simulink model "Plastic_Washer_R2020a"  (R2020a)
settings: Solver=VariableStepAuto  StartTime=0.0  StopTime=60*60*8  RelTol=1e-3  AbsTol=1e-3
libraries: fl_lib x20, nesl_utility x7, simulink x2, SimscapeFluids_lib x1
settings Model: Creator=YXL1108  LastModifiedBy=YXL1108
settings SolverCC: AutoScaleAbsTol=off
settings DebuggingCC: SymbolicDimsDataTypeCodeGenerationDiagnostic=none
settings SFSimCC: CustomCodeUndefinedFunction=UseInterfaceOnly
settings SimscapeCC: SimscapeLogType=all  SimscapeLogSimulationStatistics=on  SimscapeLogDataHistory=10000

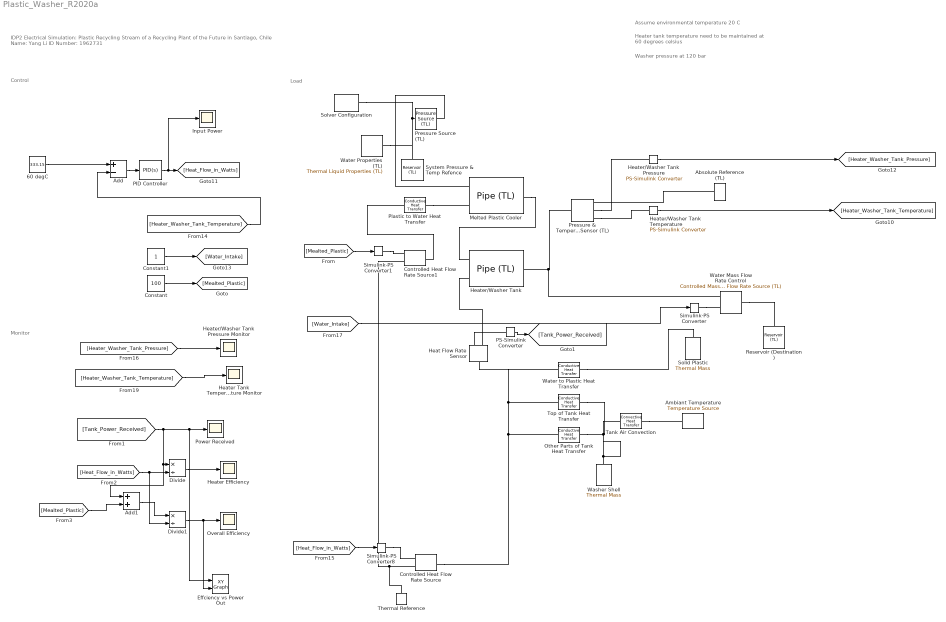
== system Plastic_Washer_R2020a ==
  note: Washer pressure at 120 bar
  note: Load
  note: Monitor
  note: Control
  note: Heater tank temperature need to be maintained at
      | 60 degrees celsius
  note: Assume environmental temperature 20 C
  note: IDP2 Electrical Simulation: Plastic Recycling Stream of a Recycling Plant of the Future in Santiago, Chile
      | Name: Yang Li
      | ID Number: 1962731
  60 degC : Constant  Value=333.15
  Absolute Reference (TL) : fl_lib/Thermal Liquid/Elements/Absolute Reference (TL)
      settings: SourceProductBaseCode=SS
  Add : Sum  Inputs=+-
  Add1 : Sum
  Ambiant Temperature : fl_lib/Thermal/Thermal Sources/Temperature Source  temperature=20 degC
  Constant : Constant  Value=100
  Constant1 : Constant
  Controlled Heat Flow Rate Source : fl_lib/Thermal/Thermal Sources/Controlled Heat Flow Rate Source
  Controlled Heat Flow Rate Source1 : fl_lib/Thermal/Thermal Sources/Controlled Heat Flow Rate Source
  Divide : Product  Inputs=*/
  Divide1 : Product  Inputs=*/
  Effciency vs Power Out : simulink/Sinks/XY Graph  xmin=1.63e+5  xmax=1.645e+5  ymin=0  ymax=1  st=-1
  Heat Flow Rate Sensor : fl_lib/Thermal/Thermal Sensors/Heat Flow Rate Sensor
      settings: SourceProductBaseCode=SS
  Heater Efficiency : Scope
  Heater Tank Temperature Monitor : Scope
  Heater/Washer Tank : fl_lib/Thermal Liquid/Elements/Pipe (TL)  length=3.5 m  area=12.25 m^2  Dh=3.5 m  length_add=1 m  roughness=15e-6 m  Re_lam=2000  Re_tur=4000  shape_factor=64  Nu_lam=3.66  dynamic_compressibility=simscape.enum.onoff.on  inertia=simscape.enum.onoff.off  p0=1 bar  T0=20 degC  mdot0=0 kg/s
      settings: SourceProductBaseCode=SS
  Heater/Washer Tank Pressure : nesl_utility/PS-Simulink Converter  PhysicalDomain=network_engine_domain  SubClassName=ps_output  LeftPortType=input  RightPortType=output  PseudoPeriodic=off  Frequencies=[]  Unit=inherit  AffineConversion=off
  Heater/Washer Tank Pressure Monitor : Scope
  Heater/Washer Tank Temperature : nesl_utility/PS-Simulink Converter  PhysicalDomain=network_engine_domain  SubClassName=ps_output  LeftPortType=input  RightPortType=output  PseudoPeriodic=off  Frequencies=[]  Unit=inherit  AffineConversion=off
  Input Power : Scope
  Melted Plastic Cooler : fl_lib/Thermal Liquid/Elements/Pipe (TL)  length=100 m  area=0.0009 m^2  Dh=0.03 m  length_add=1 m  roughness=15e-6 m  Re_lam=2000  Re_tur=4000  shape_factor=64  Nu_lam=3.66  dynamic_compressibility=simscape.enum.onoff.on  inertia=simscape.enum.onoff.off  p0=1 bar  T0=20 degC  mdot0=0 kg/s
      settings: SourceProductBaseCode=SS
  Other Parts of Tank Heat Transfer : fl_lib/Thermal/Thermal Elements/Conductive Heat Transfer  area=40 m^2  thickness=0.05 m  th_cond=45 W/(m*K)  T_specify=off  T_priority=None  T=0 K  T_nominal_specify=off  T_nominal_unit=K  T_nominal_value=1  Q_specify=off  Q_priority=None  Q=0 W  Q_nominal_specify=off  Q_nominal_unit=W  Q_nominal_value=1
  Overall Efficiency : Scope
  PID Controller : simulink/Continuous/PID Controller  Controller=PID  Form=Parallel  TimeDomain=Continuous-time  UseExternalTs=off  SampleTime=-1  IntegratorMethod=Forward Euler  FilterMethod=Forward Euler  ControllerParametersSource=internal  P=10000  I=4  D=1000000000000  UseFilter=on  N=100  TunerSelectOption=Transfer Function Based (PID Tuner App)  InitialConditionSource=internal  InitialConditionForIntegrator=0  InitialConditionForFilter=0  DifferentiatorICPrevScaledInput=0  ExternalReset=none  TrackingMode=off  Kt=1  LimitOutput=off  UpperSaturationLimit=inf  LowerSaturationLimit=-inf  LinearizeAsGain=on  AntiWindupMode=none  Kb=1  POutMin=[]  POutMax=[]  IOutMin=[]  IOutMax=[]  DOutMin=[]  DOutMax=[]  NOutMin=[]  NOutMax=[]  SumOutMin=[]  SumOutMax=[]  SaturationOutMin=[]  SaturationOutMax=[]  PParamMin=[]  PParamMax=[]  IParamMin=[]  IParamMax=[]  DParamMin=[]  DParamMax=[]  NParamMin=[]  NParamMax=[]  KbParamMin=[]  KbParamMax=[]  KtParamMin=[]  KtParamMax=[]  KbOutMin=[]  KbOutMax=[]  KtOutMin=[]  KtOutMax=[]  IntegratorOutMin=[]  IntegratorOutMax=[]  FilterOutMin=[]  FilterOutMax=[]  SumI1OutMin=[]  SumI1OutMax=[]  SumI2OutMin=[]  SumI2OutMax=[]  SumI3OutMin=[]  SumI3OutMax=[]  SumI4OutMin=[]  SumI4OutMax=[]  SumDOutMin=[]  SumDOutMax=[]  DifferentiatorOutMin=[]  DifferentiatorOutMax=[]  FilterDiffOutCoefMin=[]  FilterDiffOutCoefMax=[]  ReciprocalOutMin=[]  ReciprocalOutMax=[]  SumDenOutMin=[]  SumDenOutMax=[]  SumNumOutMin=[]  SumNumOutMax=[]  DivideOutMin=[]  DivideOutMax=[]  UdiffTsProdOutMin=[]  UdiffTsProdOutMax=[]  NTsProdOutMin=[]  NTsProdOutMax=[]  UintegralTsProdOutMin=[]  UintegralTsProdOutMax=[]  UngainTsProdOutMin=[]  UngainTsProdOutMax=[]  IntegratorContinuousStateAttributes=''  IntegratorStateMustResolveToSignalObject=off  IntegratorRTWStateStorageClass=Auto  FilterContinuousStateAttributes=''  FilterStateMustResolveToSignalObject=off  FilterRTWStateStorageClass=Auto  ParallelPVariant=InternalParameters  IdealPVariant=Disabled  IVariant=InternalParameters  DVariant=InternalParameters  IntegratorVariant=Continuous  SatVariant=Disabled  AWVariant=Passthrough  PCopyVariant=Disabled  TRVariant=Disabled  FdbkBlocksVariant=Forward  IdealPFdbkVariant=Disabled  SatFdbkVariant=Disabled  DerivativeFilterVariant=ContFilter  NVariant=InternalParameters  NCopyVariant=Disabled  FilterICVariant=InternalICsFilter  IntegratorICVariant=InternalICs  ExternalResetVariant=Disabled  TRSumVariant=Passthrough  SumFdbkVariant=Disabled  SumVariant=Sum_PID  TsampFilterVariant=InternalTs  TsampNgainVariant=Passthrough  TsampIntegralVariant=Passthrough
  PS-Simulink Converter : nesl_utility/PS-Simulink Converter  PhysicalDomain=network_engine_domain  SubClassName=ps_output  LeftPortType=input  RightPortType=output  PseudoPeriodic=off  Frequencies=[]  Unit=inherit  AffineConversion=off
  Plastic to Water Heat Transfer : fl_lib/Thermal/Thermal Elements/Conductive Heat Transfer  area=12 m^2  thickness=0.1 m  th_cond=401 W/(m*K)  T_specify=off  T_priority=None  T=0 K  T_nominal_specify=off  T_nominal_unit=K  T_nominal_value=1  Q_specify=off  Q_priority=None  Q=0 W  Q_nominal_specify=off  Q_nominal_unit=W  Q_nominal_value=1
  Power Received : Scope
  Pressure & Temperature Sensor (TL) : fl_lib/Thermal Liquid/Sensors/Pressure & Temperature Sensor (TL)
      settings: SourceProductBaseCode=SS  InternalSimscapePortConfiguration="{\"Bottom\":[],\"Left\":[{\"id\":\"A\",\"label\":\"A\",\"type\":\"foundation.thermal_liquid.thermal_liquid\"}],\"Right\":[{\"id\":\"B\",\"label\":\"B\",\"type\":\"foundation.thermal_liquid.thermal_liquid\"},{\"id\":\"P\",\"label\":\"P\",\"type\":\"output\"},{\"id\":\"T\",\"label\":\"T\",\"type\":\"output\"}],\"Top\":[]}"
  Pressure Source (TL) : fl_lib/Thermal Liquid/Sources/Pressure Source (TL)  commanded_pressure=120 bar  area=0.01 m^2
      settings: SourceProductBaseCode=SS  InternalSimscapePortConfiguration="{\"Bottom\":[],\"Left\":[{\"id\":\"A\",\"label\":\"A\",\"type\":\"foundation.thermal_liquid.thermal_liquid\"}],\"Right\":[{\"id\":\"B\",\"label\":\"B\",\"type\":\"foundation.thermal_liquid.thermal_liquid\"}],\"Top\":[]}"
  Reservoir (Destination) : fl_lib/Thermal Liquid/Elements/Reservoir (TL)  pressure_spec=foundation.enum.pressure_spec.atmospheric  reservoir_pressure=0.101325 MPa  reservoir_temperature=20 degC  area=0.01 m^2
      settings: SourceProductBaseCode=SS
  Simulink-PS Converter : nesl_utility/Simulink-PS Converter  PhysicalDomain=network_engine_domain  SubClassName=ps_input  LeftPortType=input  RightPortType=output  PseudoPeriodic=off  Frequencies=[]  NoiseDistribution=none  NoiseParameters=[]  Unit=1  AffineConversion=off  FilteringAndDerivatives=provide  SimscapeFilterOrder=1  InputFilterTimeConstant=0.001  UdotUserProvided=0
  Simulink-PS Converter1 : nesl_utility/Simulink-PS Converter  PhysicalDomain=network_engine_domain  SubClassName=ps_input  LeftPortType=input  RightPortType=output  PseudoPeriodic=off  Frequencies=[]  NoiseDistribution=none  NoiseParameters=[]  Unit=1  AffineConversion=off  FilteringAndDerivatives=provide  SimscapeFilterOrder=1  InputFilterTimeConstant=0.001  UdotUserProvided=0
  Simulink-PS Converter8 : nesl_utility/Simulink-PS Converter  PhysicalDomain=network_engine_domain  SubClassName=ps_input  LeftPortType=input  RightPortType=output  PseudoPeriodic=off  Frequencies=[]  NoiseDistribution=none  NoiseParameters=[]  Unit=1  AffineConversion=off  FilteringAndDerivatives=provide  SimscapeFilterOrder=1  InputFilterTimeConstant=0.001  UdotUserProvided=0
  Solid Plastic : fl_lib/Thermal/Thermal Elements/Thermal Mass  mass=10000 kg  sp_heat=1670 J/kg/K  T_specify=off  T_priority=High  T=300 K  T_nominal_specify=off  T_nominal_unit=K  T_nominal_value=1  Q_specify=off  Q_priority=None  Q=0 W  Q_nominal_specify=off  Q_nominal_unit=W  Q_nominal_value=1
  Solver Configuration : nesl_utility/Solver Configuration  PhysicalDomain=network_engine_domain  SubClassName=solver  LeftPortType=input  RightPortType=generic  Tones=[]  Harmonics=[]  SimulateNoise=off  Profile=off  UseLocalSampling=off  EnableSwitchedLinearOptims=on  FrequencyDomain=off  UseCCode=off  RelTol=0.001  AbsTol=1e-06  MinStep=1e-09  ToWorkspace=off  RevertToSquareIcSolve=off  NumHomotopyIterations=100  PhasorMode=off  PhasorModeNumHarmonics=1  DoDC=off  ResidualTolerance=1e-09  UseLocalSolver=off  LocalSolverChoice=NE_BACKWARD_EULER_ADVANCER  LocalSolverSampleTime=0.001  DoFixedCost=off  MaxNonlinIter=3  MaxModeIter=2  LinearAlgebra=auto  EquationFormulation=NE_TIME_EF  DelaysMemoryBudget=1024  AutomaticFiltering=on  FilteringTimeConstant=0.001  PartitionStorageMethod=AS_NEEDED  PartitionMemoryBudget=1024  PartitionMethod=ROBUST
  System Pressure & Temp Refence : fl_lib/Thermal Liquid/Elements/Reservoir (TL)  pressure_spec=foundation.enum.pressure_spec.atmospheric  reservoir_pressure=0.101325 MPa  reservoir_temperature=20 degC  area=0.01 m^2
      settings: SourceProductBaseCode=SS
  Tank Air Convection : fl_lib/Thermal/Thermal Elements/Convective Heat Transfer  area=48 m^2  heat_tr_coeff=7.9 W/(m^2 * K)  T_specify=off  T_priority=None  T=0 K  T_nominal_specify=off  T_nominal_unit=K  T_nominal_value=1  Q_specify=off  Q_priority=None  Q=0 W  Q_nominal_specify=off  Q_nominal_unit=W  Q_nominal_value=1
  Thermal Reference : fl_lib/Thermal/Thermal Elements/Thermal Reference
  Top of Tank Heat Transfer : fl_lib/Thermal/Thermal Elements/Conductive Heat Transfer  area=8 m^2  thickness=0.05 m  th_cond=60 W/(m*K)  T_specify=off  T_priority=None  T=0 K  T_nominal_specify=off  T_nominal_unit=K  T_nominal_value=1  Q_specify=off  Q_priority=None  Q=0 W  Q_nominal_specify=off  Q_nominal_unit=W  Q_nominal_value=1
  Washer Shell : fl_lib/Thermal/Thermal Elements/Thermal Mass  mass=948 kg  sp_heat=420 J/kg/K  T_specify=off  T_priority=High  T=300 K  T_nominal_specify=off  T_nominal_unit=K  T_nominal_value=1  Q_specify=off  Q_priority=None  Q=0 W  Q_nominal_specify=off  Q_nominal_unit=W  Q_nominal_value=1
  Water Properties (TL) : SimscapeFluids_lib/Thermal Liquid/Utilities/Thermal Liquid Properties (TL)  fluid_list=fluids.thermal_liquid.utilities.enum.thermal_liquid_fluid_list.water  concentration_param_EG=fluids.thermal_liquid.utilities.enum.thermal_liquid_concentration.volume_fraction  concentration_param_PG=fluids.thermal_liquid.utilities.enum.thermal_liquid_concentration.volume_fraction  c_mass_SW=3.5e-3  c_mass_EG=0.1  c_mass_PG=0.1  c_mass_GL=0.1  c_vol_EG=0.1  c_vol_PG=0.1  beta_const_EG=2.1791 GPa  beta_const_PG=2.1791 GPa  beta_const_GL=2.1791 GPa  p_min_EG=0.01 MPa  p_min_PG=0.01 MPa  p_min_GL=0.01 MPa  p_max_EG=50 MPa  p_max_PG=50 MPa  p_max_GL=50 MPa  p_atm=0.101325 MPa
      settings: SourceProductBaseCode=SH
  Water Mass Flow Rate Control : fl_lib/Thermal Liquid/Sources/Controlled Mass Flow Rate Source (TL)  area=0.0001 m^2
      settings: SourceProductBaseCode=SS  InternalSimscapePortConfiguration="{\"Bottom\":[],\"Left\":[{\"id\":\"A\",\"label\":\"A\",\"type\":\"foundation.thermal_liquid.thermal_liquid\"},{\"id\":\"M\",\"label\":\"M\",\"type\":\"input\"}],\"Right\":[{\"id\":\"B\",\"label\":\"B\",\"type\":\"foundation.thermal_liquid.thermal_liquid\"}],\"Top\":[]}"
  Water to Plastic Heat Transfer : fl_lib/Thermal/Thermal Elements/Conductive Heat Transfer  area=48 m^2  thickness=0.1 m  th_cond=401 W/(m*K)  T_specify=off  T_priority=None  T=0 K  T_nominal_specify=off  T_nominal_unit=K  T_nominal_value=1  Q_specify=off  Q_priority=None  Q=0 W  Q_nominal_specify=off  Q_nominal_unit=W  Q_nominal_value=1
  wires:
  [Water_Intake] -> Simulink-PS Converter/1
  Heater/Washer Tank Pressure/1 -> [Heater_Washer_Tank_Pressure]
  [Heat_Flow_in_Watts] -> Simulink-PS Converter8/1
  Heater/Washer Tank Temperature/1 -> [Heater_Washer_Tank_Temperature]
  Constant1/1 -> [Water_Intake]
  [Heater_Washer_Tank_Temperature] -> Heater Tank Temperature Monitor/1
  [Heater_Washer_Tank_Pressure] -> Heater/Washer Tank Pressure Monitor/1
  [Mealted_Plastic] -> Simulink-PS Converter1/1
  Constant/1 -> [Mealted_Plastic]
  60 degC/1 -> Add/1
  Add/1 -> PID Controller/1
  PID Controller/1 -> Input Power/1, [Heat_Flow_in_Watts]
  [Heater_Washer_Tank_Temperature] -> Add/2
  PS-Simulink Converter/1 -> [Tank_Power_Received]
  [Tank_Power_Received] -> Add1/1, Divide/1, Effciency vs Power Out/1, Power Received/1
  Divide/1 -> Heater Efficiency/1
  [Heat_Flow_in_Watts] -> Divide1/2, Divide/2
  Divide1/1 -> Effciency vs Power Out/2, Overall Efficiency/1
  [Mealted_Plastic] -> Add1/2
  Add1/1 -> Divide1/1
  connections:
  Controlled Heat Flow Rate Source/LConn1 -- Heat Flow Rate Sensor/LConn1 -- Water to Plastic Heat Transfer/LConn1 -- Top of Tank Heat Transfer/LConn1 -- Other Parts of Tank Heat Transfer/LConn1
  Washer Shell/LConn1 -- Tank Air Convection/LConn1 -- Top of Tank Heat Transfer/RConn1 -- Other Parts of Tank Heat Transfer/RConn1
  System Pressure & Temp Refence/LConn1 -- Water Properties (TL)/RConn1 -- Solver Configuration/RConn1 -- Pressure Source (TL)/LConn1
  Water to Plastic Heat Transfer/RConn1 -- Solid Plastic/LConn1
  Simulink-PS Converter8/RConn1 -- Controlled Heat Flow Rate Source/RConn1
  Pressure & Temperature Sensor (TL)/RConn3 -- Heater/Washer Tank Temperature/LConn1
  Melted Plastic Cooler/LConn1 -- Pressure Source (TL)/RConn1
  Melted Plastic Cooler/RConn1 -- Heater/Washer Tank/LConn1
  Absolute Reference (TL)/LConn1 -- Pressure & Temperature Sensor (TL)/RConn1
  Water Mass Flow Rate Control/RConn1 -- Reservoir (Destination)/LConn1
  Thermal Reference/LConn1 -- Controlled Heat Flow Rate Source/RConn2 -- Controlled Heat Flow Rate Source1/RConn2
  Simulink-PS Converter/RConn1 -- Water Mass Flow Rate Control/LConn2
  Plastic to Water Heat Transfer/RConn1 -- Melted Plastic Cooler/LConn2
  Pressure & Temperature Sensor (TL)/RConn2 -- Heater/Washer Tank Pressure/LConn1
  Tank Air Convection/RConn1 -- Ambiant Temperature/LConn1
  Pressure & Temperature Sensor (TL)/LConn1 -- Water Mass Flow Rate Control/LConn1 -- Heater/Washer Tank/RConn1
  Plastic to Water Heat Transfer/LConn1 -- Controlled Heat Flow Rate Source1/LConn1
  Simulink-PS Converter1/RConn1 -- Controlled Heat Flow Rate Source1/RConn1
  Heat Flow Rate Sensor/RConn2 -- Heater/Washer Tank/LConn2
  Heat Flow Rate Sensor/RConn1 -- PS-Simulink Converter/LConn1
